simulink model "MdXX_RspOutComm"  (R2022b)
settings: Solver=FixedStepDiscrete  StartTime=0.0  StopTime=10.0  FixedStep=0.01  RelTol=1e-3
undefined symbols (not defined in the file or in its folder): KeSMSuRspStatHldTm_Val, MdRspLocal2, SrcReqTp1
libraries: simulink x64, RspLib x32
(part 5 of 5)

== system MdXX_RspOutComm/MdXX_RspOutCommCalc_Cal_sys/Subsystem/MdRspOutDataSelc6/BitSelector1 ==
  U : Inport
  Bit : Inport  Port=2
  Bitwise Operator : simulink/Logic and Bit Operations/Bitwise Operator  logicop=AND  UseBitMask=off  NumInputPorts=2  BitMask=bin2dec('11011001')  BitMaskRealWorld=Stored Integer
  Constant2 : Constant  OutDataTypeStr=uint32
  Constant4 : Constant  Value=0  OutDataTypeStr=uint32
  Relational Operator : RelationalOperator  Operator=>  OutDataTypeStr=boolean  RndMeth=Simplest  InputSameDT=off
  Shift Arithmetic : ArithShift  BitShiftNumberSource=Input port  BitShiftNumber=8  BitShiftDirection=Left
      settings: InputPortMap=u0,p1
  BitOut : Outport  VectorParamsAs1DForOutWhenUnconnected=off
  wires:
  Relational Operator/1 -> BitOut/1
  Constant4/1 -> Relational Operator/2
  Constant2/1 -> Shift Arithmetic/1
  Bitwise Operator/1 -> Relational Operator/1
  U/1 -> Bitwise Operator/1
  Shift Arithmetic/1 -> Bitwise Operator/2
  Bit/1 -> Shift Arithmetic/2

== system MdXX_RspOutComm/MdXX_RspOutCommCalc_Cal_sys/Subsystem/MdRspOutDataSelc7/BitSelector ==
  U : Inport
  Bit : Inport  Port=2
  Bitwise Operator : simulink/Logic and Bit Operations/Bitwise Operator  logicop=AND  UseBitMask=off  NumInputPorts=2  BitMask=bin2dec('11011001')  BitMaskRealWorld=Stored Integer
  Constant2 : Constant  OutDataTypeStr=uint32
  Constant4 : Constant  Value=0  OutDataTypeStr=uint32
  Relational Operator : RelationalOperator  Operator=>  OutDataTypeStr=boolean  RndMeth=Simplest  InputSameDT=off
  Shift Arithmetic : ArithShift  BitShiftNumberSource=Input port  BitShiftNumber=8  BitShiftDirection=Left
      settings: InputPortMap=u0,p1
  BitOut : Outport  VectorParamsAs1DForOutWhenUnconnected=off
  wires:
  Relational Operator/1 -> BitOut/1
  Constant4/1 -> Relational Operator/2
  Constant2/1 -> Shift Arithmetic/1
  Bitwise Operator/1 -> Relational Operator/1
  U/1 -> Bitwise Operator/1
  Shift Arithmetic/1 -> Bitwise Operator/2
  Bit/1 -> Shift Arithmetic/2

== system MdXX_RspOutComm/MdXX_RspOutCommCalc_Cal_sys/Subsystem/MdRspOutDataSelc7/BitSelector1 ==
  U : Inport
  Bit : Inport  Port=2
  Bitwise Operator : simulink/Logic and Bit Operations/Bitwise Operator  logicop=AND  UseBitMask=off  NumInputPorts=2  BitMask=bin2dec('11011001')  BitMaskRealWorld=Stored Integer
  Constant2 : Constant  OutDataTypeStr=uint32
  Constant4 : Constant  Value=0  OutDataTypeStr=uint32
  Relational Operator : RelationalOperator  Operator=>  OutDataTypeStr=boolean  RndMeth=Simplest  InputSameDT=off
  Shift Arithmetic : ArithShift  BitShiftNumberSource=Input port  BitShiftNumber=8  BitShiftDirection=Left
      settings: InputPortMap=u0,p1
  BitOut : Outport  VectorParamsAs1DForOutWhenUnconnected=off
  wires:
  Bit/1 -> Shift Arithmetic/2
  Shift Arithmetic/1 -> Bitwise Operator/2
  U/1 -> Bitwise Operator/1
  Bitwise Operator/1 -> Relational Operator/1
  Constant2/1 -> Shift Arithmetic/1
  Constant4/1 -> Relational Operator/2
  Relational Operator/1 -> BitOut/1

== system MdXX_RspOutComm/MdXX_RspOutCommCalc_Cal_sys/Subsystem/MdRspOutDataSelc8/BitSelector ==
  U : Inport
  Bit : Inport  Port=2
  Bitwise Operator : simulink/Logic and Bit Operations/Bitwise Operator  logicop=AND  UseBitMask=off  NumInputPorts=2  BitMask=bin2dec('11011001')  BitMaskRealWorld=Stored Integer
  Constant2 : Constant  OutDataTypeStr=uint32
  Constant4 : Constant  Value=0  OutDataTypeStr=uint32
  Relational Operator : RelationalOperator  Operator=>  OutDataTypeStr=boolean  RndMeth=Simplest  InputSameDT=off
  Shift Arithmetic : ArithShift  BitShiftNumberSource=Input port  BitShiftNumber=8  BitShiftDirection=Left
      settings: InputPortMap=u0,p1
  BitOut : Outport  VectorParamsAs1DForOutWhenUnconnected=off
  wires:
  Bit/1 -> Shift Arithmetic/2
  Shift Arithmetic/1 -> Bitwise Operator/2
  U/1 -> Bitwise Operator/1
  Bitwise Operator/1 -> Relational Operator/1
  Constant2/1 -> Shift Arithmetic/1
  Constant4/1 -> Relational Operator/2
  Relational Operator/1 -> BitOut/1

== system MdXX_RspOutComm/MdXX_RspOutCommCalc_Cal_sys/Subsystem/MdRspOutDataSelc8/BitSelector1 ==
  U : Inport
  Bit : Inport  Port=2
  Bitwise Operator : simulink/Logic and Bit Operations/Bitwise Operator  logicop=AND  UseBitMask=off  NumInputPorts=2  BitMask=bin2dec('11011001')  BitMaskRealWorld=Stored Integer
  Constant2 : Constant  OutDataTypeStr=uint32
  Constant4 : Constant  Value=0  OutDataTypeStr=uint32
  Relational Operator : RelationalOperator  Operator=>  OutDataTypeStr=boolean  RndMeth=Simplest  InputSameDT=off
  Shift Arithmetic : ArithShift  BitShiftNumberSource=Input port  BitShiftNumber=8  BitShiftDirection=Left
      settings: InputPortMap=u0,p1
  BitOut : Outport  VectorParamsAs1DForOutWhenUnconnected=off
  wires:
  Relational Operator/1 -> BitOut/1
  Constant4/1 -> Relational Operator/2
  Constant2/1 -> Shift Arithmetic/1
  Bitwise Operator/1 -> Relational Operator/1
  U/1 -> Bitwise Operator/1
  Shift Arithmetic/1 -> Bitwise Operator/2
  Bit/1 -> Shift Arithmetic/2

== system MdXX_RspOutComm/MdXX_RspOutCommCalc_Cal_sys/Subsystem/MdRspOutDataSelc9/BitSelector ==
  U : Inport
  Bit : Inport  Port=2
  Bitwise Operator : simulink/Logic and Bit Operations/Bitwise Operator  logicop=AND  UseBitMask=off  NumInputPorts=2  BitMask=bin2dec('11011001')  BitMaskRealWorld=Stored Integer
  Constant2 : Constant  OutDataTypeStr=uint32
  Constant4 : Constant  Value=0  OutDataTypeStr=uint32
  Relational Operator : RelationalOperator  Operator=>  OutDataTypeStr=boolean  RndMeth=Simplest  InputSameDT=off
  Shift Arithmetic : ArithShift  BitShiftNumberSource=Input port  BitShiftNumber=8  BitShiftDirection=Left
      settings: InputPortMap=u0,p1
  BitOut : Outport  VectorParamsAs1DForOutWhenUnconnected=off
  wires:
  Relational Operator/1 -> BitOut/1
  Constant4/1 -> Relational Operator/2
  Constant2/1 -> Shift Arithmetic/1
  Bitwise Operator/1 -> Relational Operator/1
  U/1 -> Bitwise Operator/1
  Shift Arithmetic/1 -> Bitwise Operator/2
  Bit/1 -> Shift Arithmetic/2

== system MdXX_RspOutComm/MdXX_RspOutCommCalc_Cal_sys/Subsystem/MdRspOutDataSelc9/BitSelector1 ==
  U : Inport
  Bit : Inport  Port=2
  Bitwise Operator : simulink/Logic and Bit Operations/Bitwise Operator  logicop=AND  UseBitMask=off  NumInputPorts=2  BitMask=bin2dec('11011001')  BitMaskRealWorld=Stored Integer
  Constant2 : Constant  OutDataTypeStr=uint32
  Constant4 : Constant  Value=0  OutDataTypeStr=uint32
  Relational Operator : RelationalOperator  Operator=>  OutDataTypeStr=boolean  RndMeth=Simplest  InputSameDT=off
  Shift Arithmetic : ArithShift  BitShiftNumberSource=Input port  BitShiftNumber=8  BitShiftDirection=Left
      settings: InputPortMap=u0,p1
  BitOut : Outport  VectorParamsAs1DForOutWhenUnconnected=off
  wires:
  Bit/1 -> Shift Arithmetic/2
  Shift Arithmetic/1 -> Bitwise Operator/2
  U/1 -> Bitwise Operator/1
  Bitwise Operator/1 -> Relational Operator/1
  Constant2/1 -> Shift Arithmetic/1
  Constant4/1 -> Relational Operator/2
  Relational Operator/1 -> BitOut/1
